simulink library "HEV_Electrical_Lib"  (R2024b)
settings: Solver=ode23t  StartTime=0.0  StopTime=10  MaxStep=1e-3  RelTol=1e-3
values from neighbouring files (symbols this model uses):
  Ts = 2e-6    (= 2e-06)    [param.m]
undefined symbols (not defined in the file or in its folder): DiscIntNeverNeededParam, HEV_Param, magnitude
libraries: fl_lib x73, nesl_utility x30, spsCurrentMeasurementLib x23, spsIdealSwitchLib x12, spsVoltageMeasurementLib x11, simulink_extras x8, spsControlledCurrentSourceLib x7, spsSeriesRLCBranchLib x6, simulink x6, spsControlledVoltageSourceLib x5, spsPermanentMagnetSynchronousMachineLib x4, spsUniversalBridgeLib x3
(part 1 of 4)
Description:
  | Copyright 2008-2023 The MathWorks(TM), Inc.
settings Model: Creator=Xpatrice  LastModifiedBy=froshoo
settings SolverCC: AlgebraicLoopSolver=TrustRegion
settings DataIOCC: LimitDataPoints=on  SaveFormat=Array  SignalLoggingSaveFormat=ModelDataLogs  ReturnWorkspaceOutputs=off
settings OptimizationCC: BlockReduction=off  BooleanDataType=off  ReuseModelBlockBuffer=off  ExpressionDepthLimit=2147483647  LifeSpan=inf
settings DebuggingCC: SaveWithParameterizedLinksMsg=none  UnderspecifiedInitializationDetection=Classic  MergeDetectMultiDrivingBlocksExec=none  SignalResolutionControl=TryResolveAllWithWarning  FcnCallInpInsideContextMsg=warning  UnconnectedInputMsg=warning  UnconnectedOutputMsg=warning  UnconnectedLineMsg=warning  AllowSymbolicDim=off  StateNameClashWarn=warning  PregeneratedLibrarySubsystemCodeDiagnostic=none  SFUnexpectedBacktrackingDiag=warning  SFNoUnconditionalDefaultTransitionDiag=warning  SFExecutionAtInitializationDiag=none  ArithmeticOperatorsInVariantConditions=warning
settings HardwareCC: ProdBitPerPointer=32  ProdBitPerSizeT=32  ProdBitPerPtrDiffT=32  ProdLargestAtomicFloat=None  ProdIntDivRoundTo=Undefined  ProdEndianess=Unspecified  ProdWordSize=32  ProdHWDeviceType=32-bit Generic  TargetUnknown=on
settings ModelReferenceCC: EnableRefExpFcnMdlSchedulingChecks=on  PropagateSignalLabelsOutOfModel=off
settings SFSimCC: SimUseLocalCustomCode=off  CustomCodeUndefinedFunction=UseInterfaceOnly
settings RTWCC: RTWUseLocalCustomCode=off  GPUComputeCapability=3.5  DLArmComputeVersion=19.05
settings CodeAppCC: StateflowObjectComments=on
settings GRTTargetCC: TargetLangStandard=C89/C90 (ANSI)  CombineOutputUpdateFcns=off  GRTInterface=on
settings ConfigComp: CovMetricSettings=dw  CovSaveCumulativeToWorkspaceVar=on  CovSaveSingleToWorkspaceVar=on  CovExternalEMLEnable=off  CovSFcnEnable=off

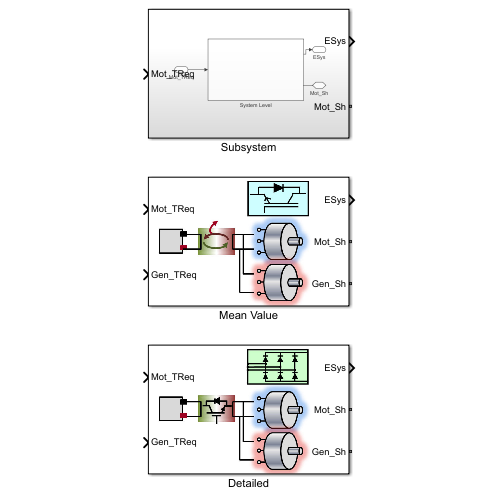
[thumbnail: Simulink's stored preview of the top-level diagram]
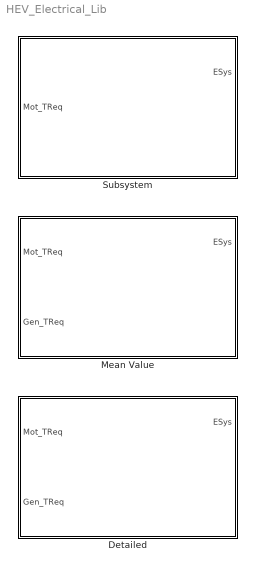
== system HEV_Electrical_Lib ==
  Detailed : Subsystem  mask{popup_batteryvariant=Predefined}
      mask prompts: popup_batteryvariant "Battery Model"
      mask init:
      | set_param([gcb '/Battery'],'LabelModeActiveChoice',get_param(gcb,'popup_batteryvariant'));
      mask TypeOptions popup_batteryvariant: Predefined | Generic
      mask Display: image('HEV_Electrical_Detailed_IMAGE.jpg');
  Mean Value : Subsystem  mask{popup_batteryvariant=Predefined}
      mask prompts: popup_batteryvariant "Battery Model"
      mask init:
      | set_param([gcb '/Battery'],'LabelModeActiveChoice',get_param(gcb,'popup_batteryvariant'));
      mask TypeOptions popup_batteryvariant: Predefined | Generic
      mask Display: image('HEV_Electrical_Mean_Value_IMAGE.jpg');
  Subsystem : Subsystem

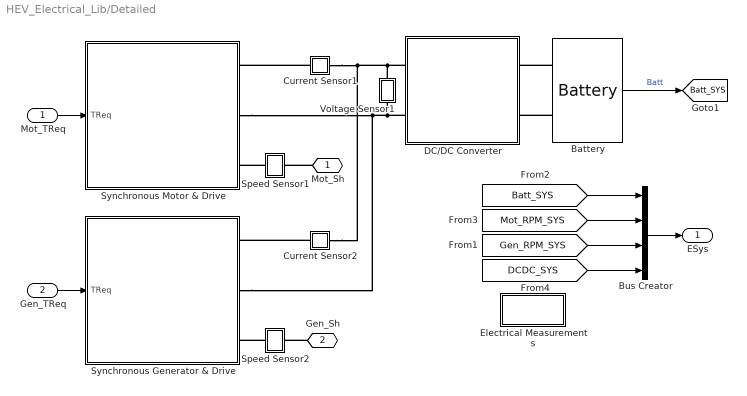
== system HEV_Electrical_Lib/Detailed ==
  Mot_TReq : Inport
  Gen_TReq : Inport  Port=2
  Battery : HEV_Battery_Det_Lib/Battery  SystemSampleTime=-1  LabelModeActiveChoice=Predefined  VariantActivationTime=update diagram  AllowFlexibleInterface=on  Latency=0  AutoFrameSizeCalculation=off
  Bus Creator : BusCreator  Inputs='Batt','Mot_RPM','Gen_RPM','DCDC_Temp'
  Current Sensor1 : Subsystem
  Current Sensor2 : Subsystem
  DC/DC Converter : Subsystem
      mask Display:
      | image(imread('HEV_DCDC_Switching_IMAGE.jpg'));
      | port_label('RConn',1,'Bus+');
      | port_label('RConn',2,'Bus-');
      | port_label('LConn',1,'Batt+');
      | port_label('LConn',2,'Batt-');
      | text(0.05,0.5,'Out');
      | text(0.85,0.5,'In');
  Electrical Measurements : Subsystem
  Speed Sensor1 : Subsystem
      mask Display: disp('S');
  Speed Sensor2 : Subsystem
      mask Display: disp('S');
  Synchronous Generator & Drive : Subsystem
      mask Display:
      | image(imread('HEV_Detailed_Generator_IMAGE.jpg'));
      | port_label('input',1,'T_Req');
      | port_label('RConn',1,'+');
      | port_label('RConn',2,'-');
      | port_label('RConn',3,'Shaft');
  Synchronous Motor & Drive : Subsystem
      mask Display:
      | image(imread('HEV_Detailed_Motor_IMAGE.jpg'));
      | port_label('input',1,'T_Req');
      | port_label('RConn',1,'+');
      | port_label('RConn',2,'-');
      | port_label('RConn',3,'Shaft');
  Voltage Sensor1 : Subsystem
  Mot_Sh : PMIOPort  Side=Right
  Gen_Sh : PMIOPort  Port=2  Side=Right
  ESys : Outport  VectorParamsAs1DForOutWhenUnconnected=off
  tag scope: Batt_SYS=global
  wires:
  [DCDC_SYS] -> Bus Creator/4
  [Batt_SYS] -> Bus Creator/1
  Bus Creator/1 -> ESys/1
  [Gen_RPM_SYS] -> Bus Creator/3
  [Mot_RPM_SYS] -> Bus Creator/2
  Gen_TReq/1 -> Synchronous Generator & Drive/1(TReq)
  Battery/1 -> [Batt_SYS]  "Batt"
  Mot_TReq/1 -> Synchronous Motor & Drive/1(TReq)
  connections:
  Gen_Sh/RConn1 -- Speed Sensor2/RConn1
  Speed Sensor2/LConn1 -- Synchronous Generator & Drive/RConn3
  Mot_Sh/RConn1 -- Speed Sensor1/RConn1
  Speed Sensor1/LConn1 -- Synchronous Motor & Drive/RConn3
  Current Sensor1/LConn1 -- Synchronous Motor & Drive/RConn1
  Current Sensor2/LConn1 -- Synchronous Generator & Drive/RConn1
  Battery/LConn2 -- DC/DC Converter/LConn2
  Battery/LConn1 -- DC/DC Converter/LConn1
  DC/DC Converter/RConn1 -- Current Sensor2/RConn1 -- Current Sensor1/RConn1 -- Voltage Sensor1/RConn1
  DC/DC Converter/RConn2 -- Synchronous Motor & Drive/RConn2 -- Synchronous Generator & Drive/RConn2 -- Voltage Sensor1/LConn1

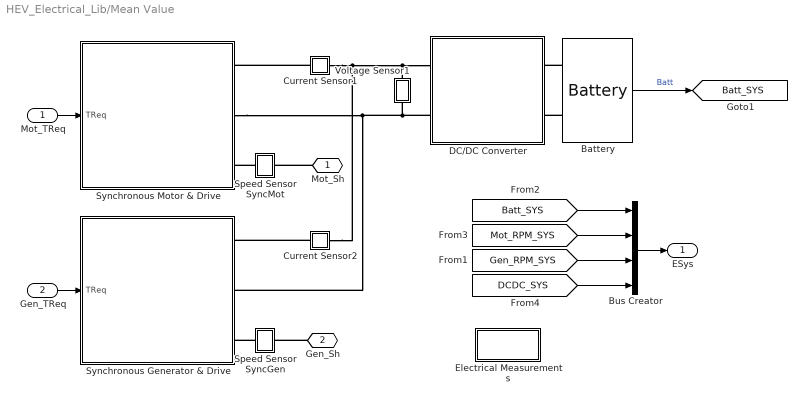
== system HEV_Electrical_Lib/Mean Value ==
  Mot_TReq : Inport
  Gen_TReq : Inport  Port=2
  Battery : HEV_Battery_Det_Lib/Battery  SystemSampleTime=-1  LabelModeActiveChoice=Predefined  VariantActivationTime=update diagram  AllowFlexibleInterface=on  Latency=0  AutoFrameSizeCalculation=off
  Bus Creator : BusCreator  Inputs='Batt','Mot_RPM','Gen_RPM','DCDC_Temp'
  Current Sensor1 : Subsystem
  Current Sensor2 : Subsystem
  DC/DC Converter : Subsystem
      mask init:
      | [X1,X1m,X2,X2m,X3,X4,Y1,Y1m,Y2,Y2m,Y3,Y4,color1,color2]=spsdrivelogo;
      mask Display:
      | image(imread('HEV_DCDC_System_IMAGE.jpg'));
      | port_label('RConn',1,'Bus+');
      | port_label('RConn',2,'Bus-');
      | port_label('LConn',1,'Batt+');
      | port_label('LConn',2,'Batt-');
      | text(0.05,0.5,'Out');
      | text(0.85,0.5,'In');
      | text(0.4,0.925,'Loss');
  Electrical Measurements : Subsystem
  Speed Sensor SyncGen : Subsystem
      mask Display: disp('S');
  Speed Sensor SyncMot : Subsystem
      mask Display: disp('S');
  Synchronous Generator & Drive : Subsystem
      mask Display:
      | image(imread('HEV_MeanValue_Generator_IMAGE.jpg'));
      | port_label('input',1,'T_Req');
      | port_label('RConn',1,'+');
      | port_label('RConn',2,'-');
      | port_label('RConn',3,'Shaft');
  Synchronous Motor & Drive : Subsystem
      mask Display:
      | image(imread('HEV_MeanValue_Motor_IMAGE.jpg'));
      | port_label('input',1,'T_Req');
      | port_label('RConn',1,'+');
      | port_label('RConn',2,'-');
      | port_label('RConn',3,'Shaft');
  Voltage Sensor1 : Subsystem
  Mot_Sh : PMIOPort  Side=Right
  Gen_Sh : PMIOPort  Port=2  Side=Right
  ESys : Outport  VectorParamsAs1DForOutWhenUnconnected=off
  tag scope: Batt_SYS=global
  wires:
  [DCDC_SYS] -> Bus Creator/4
  [Batt_SYS] -> Bus Creator/1
  Bus Creator/1 -> ESys/1
  [Gen_RPM_SYS] -> Bus Creator/3
  [Mot_RPM_SYS] -> Bus Creator/2
  Gen_TReq/1 -> Synchronous Generator & Drive/1(TReq)
  Battery/1 -> [Batt_SYS]  "Batt"
  Mot_TReq/1 -> Synchronous Motor & Drive/1(TReq)
  connections:
  Gen_Sh/RConn1 -- Speed Sensor SyncGen/RConn1
  Speed Sensor SyncGen/LConn1 -- Synchronous Generator & Drive/RConn3
  Mot_Sh/RConn1 -- Speed Sensor SyncMot/RConn1
  Speed Sensor SyncMot/LConn1 -- Synchronous Motor & Drive/RConn3
  Battery/LConn2 -- DC/DC Converter/LConn2
  Battery/LConn1 -- DC/DC Converter/LConn1
  Current Sensor2/RConn1 -- Current Sensor1/RConn1 -- DC/DC Converter/RConn1 -- Voltage Sensor1/RConn1
  DC/DC Converter/RConn2 -- Synchronous Generator & Drive/RConn2 -- Synchronous Motor & Drive/RConn2 -- Voltage Sensor1/LConn1
  Current Sensor1/LConn1 -- Synchronous Motor & Drive/RConn1
  Current Sensor2/LConn1 -- Synchronous Generator & Drive/RConn1

== system HEV_Electrical_Lib/Subsystem ==
  Mot_TReq : Inport
  System Level : Subsystem  mask{popup_batteryvariant=Predefined}
      mask prompts: popup_batteryvariant "Battery Variant"
      mask init:
      | set_param([gcb '/Battery'],'LabelModeActiveChoice',get_param(gcb,'popup_batteryvariant'));
      mask TypeOptions popup_batteryvariant: Predefined | Generic | Cells
      mask Display: image('HEV_Electrical_System_Level_IMAGE.jpg');
  Mot_Sh : PMIOPort  Side=Right
  ESys : Outport
  wires:
  Mot_TReq/1 -> System Level/1(Mot_TReq)
  System Level/1(ESys) -> ESys/1
  connections:
  System Level/RConn1 -- Mot_Sh/RConn1

== system HEV_Electrical_Lib/Detailed/Current Sensor1 ==
  i1 : spsCurrentMeasurementLib/Current Measurement  PhasorSimulation=off  OutputType=Complex  PSBequivalent=0
  - : PMIOPort  Side=Left
  + : PMIOPort  Tag=PMCPort  Port=2  Side=Right
  tag scope: Mot_Current_SYS=global
  wires:
  i1/1 -> [Mot_Current_SYS]
  connections:
  -/RConn1 -- i1/RConn1
  +/RConn1 -- i1/LConn1

== system HEV_Electrical_Lib/Detailed/Current Sensor2 ==
  i1 : spsCurrentMeasurementLib/Current Measurement  PhasorSimulation=off  OutputType=Complex  PSBequivalent=0
  + : PMIOPort  Side=Right
  - : PMIOPort  Port=2  Side=Left
  tag scope: Gen_Current_SYS=global
  wires:
  i1/1 -> [Gen_Current_SYS]
  connections:
  +/RConn1 -- i1/LConn1
  -/RConn1 -- i1/RConn1

== system HEV_Electrical_Lib/Detailed/DC//DC Converter ==
  CBus : spsSeriesRLCBranchLib/Series RLC Branch  LConnTagsString=__new0  RConnTagsString=__new0  BranchType=RC  Resistance=0.1  Inductance=1e-3  SetiL0=off  InitialCurrent=0  Capacitance=1130e-6  Setx0=on  InitialVoltage=500  Measurements=None
  CBus1 : spsSeriesRLCBranchLib/Series RLC Branch  LConnTagsString=__new0  RConnTagsString=__new0  BranchType=C  Resistance=0.2  Inductance=1e-3  SetiL0=off  InitialCurrent=0  Capacitance=282e-6  Setx0=on  InitialVoltage=150  Measurements=None
  Detailed Boost converter : spsUniversalBridgeLib/Universal Bridge  Arms=1  SnubberResistance=5000  SnubberCapacitance=inf  Device=IGBT / Diodes  Ron=1e-3  Lon=0  ForwardVoltages=[0,0]  ForwardVoltage=0  GTOparameters=[ 10e-6 , 20e-6 ]  IGBTparameters=[0,0]  Measurements=None  Measurements_2=None  converterType=Rectifier
  L : spsSeriesRLCBranchLib/Series RLC Branch  LConnTagsString=__new0  RConnTagsString=__new0  BranchType=L  Resistance=0.3  Inductance=373e-6  SetiL0=off  InitialCurrent=100  Capacitance=100e-6  Setx0=off  InitialVoltage=0  Measurements=None
  PWM : Subsystem
  Ubus Ref : Constant  Value=HEV_Param.DCDCConv.Output_Voltage
  V1 : spsVoltageMeasurementLib/Voltage Measurement  PhasorSimulation=off  OutputType=Complex  PSBequivalent=0
  Voltage Controller : Subsystem  mask(PI controller){Kp=0.001, Ki=1, Ts=Ts}
      mask prompts: Kp "Proportional gain (Kp)"; Ki "Integral gain (Ki)"; Ts "Sample time (s) :"
      mask help: Proportional-Integral Speed Controller
      mask Display: plot(0,0,100,100,[35,35,65],[70,30,30],[35,65],[45,60])
  Bus+ : PMIOPort  Tag=PMCPort  Side=Right
  Bus- : PMIOPort  Tag=PMCPort  Port=2  Side=Right
  Batt+ : PMIOPort  Tag=PMCPort  Port=3  Side=Left
  Batt- : PMIOPort  Tag=PMCPort  Port=4  Side=Left
  wires:
  PWM/1(Pulses) -> Detailed Boost converter/1
  Voltage Controller/1(Ec) -> PWM/1(Ref.)
  Ubus Ref/1 -> Voltage Controller/1(Uref)
  V1/1 -> Voltage Controller/2(UBus)
  connections:
  L/LConn1 -- Detailed Boost converter/LConn1
  Detailed Boost converter/RConn1 -- CBus/LConn1 -- V1/LConn1 -- Bus+/RConn1
  Batt+/RConn1 -- L/RConn1 -- CBus1/LConn1
  Detailed Boost converter/RConn2 -- Bus-/RConn1 -- CBus/RConn1 -- V1/LConn2 -- Batt-/RConn1 -- CBus1/RConn1

== system HEV_Electrical_Lib/Detailed/Electrical Measurements ==
  Bus Selector : BusSelector  OutputSignals=Voltage (V),Current (A),SOC (%)
  Mux : Mux  Inputs=2
  Mux1 : Mux  Inputs=3
  Mux2 : Mux  Inputs=3
  Mux3 : Mux
  Mux4 : Mux  Inputs=2
  Product1 : Product  RndMeth=Zero
  Product2 : Product  RndMeth=Zero
  Product3 : Product  RndMeth=Zero
  tag scope: Electricals=global, Power=global
  wires:
  Product2/1 -> Mux1/1  "Motor Power (W)"
  Product1/1 -> Mux1/2  "Generator power (W)"
  Product3/1 -> Mux1/3  "Battery power (W)"
  [Mot_Current_SYS] -> Product2/1, Mux2/1
  Mux1/1 -> [Power]
  [Batt_Measures] -> Bus Selector/1
  Bus Selector/1 -> Mux/2, Product3/1  "<Voltage (V)>"
  Bus Selector/2 -> Product3/2, Mux2/2  "<Current (A)>"
  Mux/1 -> Mux3/2  "Voltage (DC bus, Battery)"
  Mux2/1 -> Mux3/3  "Current (Motor, Battery, Generator)"
  [Gen_Current_SYS] -> Product1/1, Mux2/3
  Bus Selector/3 -> Mux3/4  "<SOC (%)>"
  [DC_Bus_SYS] -> Product2/2, Product1/2, Mux/1, Mux4/1, Mux4/2
  Mux3/1 -> [Electricals]
  Mux4/1 -> Mux3/1

== system HEV_Electrical_Lib/Detailed/Speed Sensor1 ==
  Ideal Rotational Motion Sensor : fl_lib/Mechanical/Mechanical Sensors/Ideal Rotational Motion Sensor  reference=foundation.enum.MeasurementReference.difference  acceleration_port=false  velocity_port=true  position_port=true  wrap_angle=simscape.enum.onoff.off  offset=0 rad
  Mechanical Rotational Reference : fl_lib/Mechanical/Rotational Elements/Mechanical Rotational Reference
  PS-Simulink Converter : nesl_utility/PS-Simulink Converter  PhysicalDomain=network_engine_domain  SubClassName=ps_output  LeftPortType=input  RightPortType=output  PseudoPeriodic=off  Frequencies=[]  VectorFormat=1-D array  Unit=rpm  AffineConversion=off
  Solver Configuration : nesl_utility/Solver Configuration  PhysicalDomain=network_engine_domain  SubClassName=solver  LeftPortType=input  RightPortType=generic  Tones=[]  Harmonics=[]  SimulateNoise=off  Profile=off  UseLocalSampling=off  EnableSwitchedLinearOptims=on  FrequencyDomain=off  UseCCode=off  RelTol=0.001  AbsTol=0.001  MinStep=1e-09  ToWorkspace=off  RevertToSquareIcSolve=off  NumHomotopyIterations=100  PhasorMode=off  PhasorModeNumHarmonics=1  ConsistencySolver=NEWTON_XTOL_AFTER_FTOL  IndexReductionMethod=DerivativeReplacement  DoDC=off  ResidualTolerance=1e-09  ConsistencyTolSource=GLOBAL  ConsistencyAbsTol=0.001  ConsistencyRelTol=0.001  ConsistencyTolFactor=0.001  UseLocalSolver=off  LocalSolverChoice=NE_BACKWARD_EULER_ADVANCER  ResolveIndetEquations=on  FunctionEvalNumThread=1  LocalSolverSampleTime=0.001  DoFixedCost=off  MaxNonlinIter=3  MaxModeIter=2  ComputeImpulses=off  ImpulseIterations=2  LinearAlgebra=auto  LinearAlgebraNumThread=0  EquationFormulation=NE_TIME_EF  DelaysMemoryBudget=1024  AutomaticFiltering=on  FilteringTimeConstant=0.001  PartitionStorageMethod=AS_NEEDED  PartitionMemoryBudget=1024  PartitionMethod=ROBUST  MultibodyUseLocalSolver=off  MultibodyLocalSolverChoice=ODE1  MultibodyLocalSolverSampleTime=0.001
  Sh : PMIOPort  Side=Left
  Sh1 : PMIOPort  Port=2  Side=Right
  tag scope: Mot_RPM_SYS=global
  wires:
  PS-Simulink Converter/1 -> [Mot_RPM_SYS]  "Mot_RPM"
  connections:
  Ideal Rotational Motion Sensor/RConn1 -- Mechanical Rotational Reference/LConn1
  Sh1/RConn1 -- Solver Configuration/RConn1 -- Ideal Rotational Motion Sensor/LConn1 -- Sh/RConn1
  PS-Simulink Converter/LConn1 -- Ideal Rotational Motion Sensor/RConn2

== system HEV_Electrical_Lib/Detailed/Speed Sensor2 ==
  Ideal Rotational Motion Sensor : fl_lib/Mechanical/Mechanical Sensors/Ideal Rotational Motion Sensor  reference=foundation.enum.MeasurementReference.difference  acceleration_port=false  velocity_port=true  position_port=true  wrap_angle=simscape.enum.onoff.off  offset=0 rad
  Mechanical Rotational Reference : fl_lib/Mechanical/Rotational Elements/Mechanical Rotational Reference
  PS-Simulink Converter : nesl_utility/PS-Simulink Converter  PhysicalDomain=network_engine_domain  SubClassName=ps_output  LeftPortType=input  RightPortType=output  PseudoPeriodic=off  Frequencies=[]  VectorFormat=1-D array  Unit=rpm  AffineConversion=off
  Solver Configuration : nesl_utility/Solver Configuration  PhysicalDomain=network_engine_domain  SubClassName=solver  LeftPortType=input  RightPortType=generic  Tones=[]  Harmonics=[]  SimulateNoise=off  Profile=off  UseLocalSampling=off  EnableSwitchedLinearOptims=on  FrequencyDomain=off  UseCCode=off  RelTol=0.001  AbsTol=0.001  MinStep=1e-09  ToWorkspace=off  RevertToSquareIcSolve=off  NumHomotopyIterations=100  PhasorMode=off  PhasorModeNumHarmonics=1  ConsistencySolver=NEWTON_XTOL_AFTER_FTOL  IndexReductionMethod=DerivativeReplacement  DoDC=off  ResidualTolerance=1e-09  ConsistencyTolSource=GLOBAL  ConsistencyAbsTol=0.001  ConsistencyRelTol=0.001  ConsistencyTolFactor=0.001  UseLocalSolver=off  LocalSolverChoice=NE_BACKWARD_EULER_ADVANCER  ResolveIndetEquations=on  FunctionEvalNumThread=1  LocalSolverSampleTime=0.001  DoFixedCost=off  MaxNonlinIter=3  MaxModeIter=2  ComputeImpulses=off  ImpulseIterations=2  LinearAlgebra=auto  LinearAlgebraNumThread=0  EquationFormulation=NE_TIME_EF  DelaysMemoryBudget=1024  AutomaticFiltering=on  FilteringTimeConstant=0.001  PartitionStorageMethod=AS_NEEDED  PartitionMemoryBudget=1024  PartitionMethod=ROBUST  MultibodyUseLocalSolver=off  MultibodyLocalSolverChoice=ODE1  MultibodyLocalSolverSampleTime=0.001
  Sh : PMIOPort  Side=Left
  Sh1 : PMIOPort  Port=2  Side=Right
  tag scope: Gen_RPM_SYS=global
  wires:
  PS-Simulink Converter/1 -> [Gen_RPM_SYS]  "Gen_RPM"
  connections:
  Ideal Rotational Motion Sensor/RConn1 -- Mechanical Rotational Reference/LConn1
  PS-Simulink Converter/LConn1 -- Ideal Rotational Motion Sensor/RConn2
  Sh1/RConn1 -- Sh/RConn1 -- Solver Configuration/RConn1 -- Ideal Rotational Motion Sensor/LConn1

== system HEV_Electrical_Lib/Detailed/Synchronous Generator & Drive ==
  note: This block is based on the AC6
      | drive block
  TReq : Inport
  Bus Selector : BusSelector  OutputSignals=Rotor angle thetam (rad)
  GF : Subsystem
      mask Display: disp('GF')
  Measures : Subsystem
      settings: LibrarySourceBlock=electricdrivelib/AC drives/PM Synchronous Motor Drive/Measures
  Mux : Subsystem
  Permanent Magnet Synchronous Machine : spsPermanentMagnetSynchronousMachineLib/Permanent Magnet Synchronous Machine  NbPhases=3  FluxDistribution=Sinusoidal  RotorType=Salient-pole  MechanicalLoad=Speed w  PresetModel=No  ShowDetailedParameters=on  MeasurementBus=off  Resistance=HEV_Param.Generator.Stator_Resistance  Inductance=0  dqInductances=HEV_Param.Generator.Inductances  La=0.000835  MachineConstant=Flux linkage established by magnets (V.s)  Flux=0.192  VoltageCst=34.8249  TorqueCst=0.288  Flat=0  Mechanical=[0.011 0.001889/4 4/4]  PolePairs=1  InitialConditions=[0,0, 0,0,0]  InitialConditions5ph=[0 0 0 0 0 0]  RefAngle=90 degrees behind phase A axis (modified Park)  IterativeDiscreteModel=Trapezoidal non iterative  TsBlock=-1  TsPowergui=0
      settings: AttributesFormatString=\n
  Shaft Inertia : fl_lib/Mechanical/Rotational Elements/Inertia  inertia=HEV_Param.Generator.Shaft_Inertia kg*m^2  num_ports=foundation.enum.numPorts2.one  w_specify=on  w_priority=High  w=0 rad/s  w_nominal_specify=off  w_nominal_value=1  w_nominal_unit=rad/s  t_specify=off  t_priority=High  t=0 N*m  t_nominal_specify=off  t_nominal_value=1  t_nominal_unit=N*m
  Subsystem : Subsystem
      mask Display: disp('GF');
  Subsystem1 : Subsystem
  Three-phase Inverter : spsUniversalBridgeLib/Universal Bridge  Arms=3  SnubberResistance=5000  SnubberCapacitance=inf  Device=IGBT / Diodes  Ron=1e-3  Lon=0  ForwardVoltages="[  0  0  ]"  ForwardVoltage=0  GTOparameters=[ 10e-6 , 20e-6 ]  IGBTparameters=[ 1e-6 , 2e-6 ]*0  Measurements=None  Measurements_2=None  converterType=Rectifier
  VECT : Subsystem  mask(VECT){nb_p=1, lambda=0.192, freq_max=20e3, Ts_vect=20e-6, h=0.1}
      mask prompts: nb_p "Motor pairs of poles"; lambda "Flux induced by magnets (Wb)"; freq_max "Maximum switching frequency (Hz)"; Ts_vect "Sampling time (s)"; h "Current hysteresis bandwidth (A)"
      mask help: This block implements a vector controller.
      mask init:
      | load spsdrivelogodata.mat
      mask Display:
      | patch([spsdrivelogodata.X1 spsdrivelogodata.X1m],[spsdrivelogodata.Y1 spsdrivelogodata.Y1m],spsdrivelogodata.color1);
      | patch(spsdrivelogodata.X3,spsdrivelogodata.Y3,spsdrivelogodata.color2);
      | plot([spsdrivelogodata.X1 spsdrivelogodata.X1m spsdrivelogodata.X2 spsdrivelogodata.X2m spsdrivelogodata.X3 spsdrivelogodata.X4],[spsdrivelogodata.Y1 spsdrivelogodata.Y1m spsdrivelogodata.Y2 spsdrivelogodata.Y2m spsdrivelogodata.Y3 spsdrivelogodata.Y4]);
  + : PMIOPort  Side=Right
  - : PMIOPort  Port=2  Side=Right
  Gen_Sh : PMIOPort  Port=3  Side=Right
  wires:
  TReq/1 -> GF/1(In1)
  Bus Selector/1 -> VECT/2(teta)  "<Rotor angle thetam (rad)>"
  Mux/1(g) -> Three-phase Inverter/1
  VECT/1(gates) -> Mux/1(gates)
  Measures/1(I_abc) -> VECT/3(I_abc)
  Permanent Magnet Synchronous Machine/1 -> Bus Selector/1, Mux/2(m), Subsystem/1(In)
  Subsystem/1(Out) -> Subsystem1/1(Sig)
  Subsystem1/1(Spd) -> Permanent Magnet Synchronous Machine/1
  GF/1(Out1) -> VECT/1(Torque*)
  connections:
  Three-phase Inverter/LConn3 -- Measures/LConn3
  Measures/LConn2 -- Three-phase Inverter/LConn2
  Three-phase Inverter/LConn1 -- Measures/LConn1
  Measures/RConn3 -- Permanent Magnet Synchronous Machine/LConn3
  Measures/RConn2 -- Permanent Magnet Synchronous Machine/LConn2
  Measures/RConn1 -- Permanent Magnet Synchronous Machine/LConn1
  +/RConn1 -- Three-phase Inverter/RConn1
  -/RConn1 -- Three-phase Inverter/RConn2
  Subsystem1/RConn1 -- Gen_Sh/RConn1 -- Shaft Inertia/LConn1

== system HEV_Electrical_Lib/Detailed/Synchronous Motor & Drive ==
  note: This block is based on the
      | AC6 IPMSM drive block
  TReq : Inport
  500 Vdc 50kW PMSM : spsPermanentMagnetSynchronousMachineLib/Permanent Magnet Synchronous Machine  NbPhases=3  FluxDistribution=Sinusoidal  RotorType=Salient-pole  MechanicalLoad=Speed w  PresetModel=No  ShowDetailedParameters=on  MeasurementBus=off  Resistance=HEV_Param.Motor.Stator_Resistance  Inductance=0  dqInductances=HEV_Param.Motor.Inductances  La=0.000835  MachineConstant=Flux linkage established by magnets (V.s)  Flux=0.175666143629361  VoltageCst=127.4493  TorqueCst=1.054  Flat=0  Mechanical=[0.089 0.005 4]  PolePairs=4  InitialConditions=[0,0,0,0]  InitialConditions5ph=[0 0 0 0 0 0]  RefAngle=90 degrees behind phase A axis (modified Park)  IterativeDiscreteModel=Trapezoidal non iterative  TsBlock=-1  TsPowergui=0
      settings: AttributesFormatString=\n
  Bus Selector : BusSelector  OutputSignals=Rotor speed wm (rad/s),Rotor angle thetam (rad)
  GF : Subsystem
      mask Display: disp('GF')
  Measures : Subsystem
      settings: LibrarySourceBlock=electricdrivelib/AC drives/PM Synchronous Motor Drive/Measures
  Mux : Subsystem
  Shaft Inertia : fl_lib/Mechanical/Rotational Elements/Inertia  inertia=HEV_Param.Motor.Shaft_Inertia kg*m^2  num_ports=foundation.enum.numPorts2.one  w_specify=on  w_priority=High  w=0 rad/s  w_nominal_specify=off  w_nominal_value=1  w_nominal_unit=rad/s  t_specify=off  t_priority=High  t=0 N*m  t_nominal_specify=off  t_nominal_value=1  t_nominal_unit=N*m
  Subsystem : Subsystem
      mask Display: disp('GF');
  Subsystem1 : Subsystem
  Three-Phase Inverter : spsUniversalBridgeLib/Universal Bridge  Arms=3  SnubberResistance=5000  SnubberCapacitance=inf  Device=IGBT / Diodes  Ron=1e-3  Lon=0  ForwardVoltages="[  0  0  ]"  ForwardVoltage=0  GTOparameters=[ 10e-6 , 20e-6 ]  IGBTparameters=[ 1e-6 , 2e-6 ]*0  Measurements=None  Measurements_2=None  converterType=Rectifier
  Torque limitation : Subsystem
      mask Display: plot([0;1800;2000;2500;3000;3500], [1;1;0.90*1;0.72*1;0.6*1;0.51*1])
  VECT Controller : Subsystem  mask(VECT){nb_p=4, dqInductances=HEV_Param.Motor.Inductances, lambda=0.175666143629361, freq_max=20e3, Ts_vect=20e-6, h=0.1}
      mask prompts: nb_p "Motor pairs of poles"; dqInductances "Inductances [ Ld(H) Lq(H) ]:"; lambda "Flux induced by magnets (Wb)"; freq_max "Maximum switching frequency (Hz)"; Ts_vect "Sampling time (s)"; h "Current hysteresis bandwidth (A)"
      mask help: This block implements a vector controller.
      mask init:
      | load spsdrivelogodata.mat
      | ib = lambda/(dqInductances(2)-dqInductances(1));
      | Teb = 3/2*nb_p*lambda*ib;
      | Ld = dqInductances(1);
      | Lq = dqInductances(2);
      | lam = lambda;
      | p=nb_p;
      | ib = lam/(Lq-Ld);
      | iqn = 0:0.01:3;
      | ten = iqn/2.*(sqrt(4*iqn.*iqn+1)+1);
      mask Display:
      | patch([spsdrivelogodata.X1 spsdrivelogodata.X1m],[spsdrivelogodata.Y1 spsdrivelogodata.Y1m],spsdrivelogodata.color1);
      | patch(spsdrivelogodata.X3,spsdrivelogodata.Y3,spsdrivelogodata.color2);
      | plot([spsdrivelogodata.X1 spsdrivelogodata.X1m spsdrivelogodata.X2 spsdrivelogodata.X2m spsdrivelogodata.X3 spsdrivelogodata.X4],[spsdrivelogodata.Y1 spsdrivelogodata.Y1m spsdrivelogodata.Y2 spsdrivelogodata.Y2m spsdrivelogodata.Y3 spsdrivelogodata.Y4]);
  + : PMIOPort  Side=Right
  - : PMIOPort  Port=2  Side=Right
  Mot_Sh : PMIOPort  Port=3  Side=Right
  wires:
  TReq/1 -> GF/1(In1)
  Torque limitation/1(torque) -> VECT Controller/1(Torque*)
  Bus Selector/2 -> VECT Controller/3(teta)  "<Rotor angle thetam (rad)>"
  Measures/1(I_abc) -> VECT Controller/4(I_abc)
  Bus Selector/1 -> Torque limitation/1(N rad/s), VECT Controller/2(w)  "<Rotor speed wm (rad/s)>"
  500 Vdc 50kW PMSM/1 -> Bus Selector/1, Mux/2(m), Subsystem/1(In)
  VECT Controller/1(gates) -> Mux/1(gates)
  Mux/1(g) -> Three-Phase Inverter/1
  Subsystem/1(Out) -> Subsystem1/1(Sig)
  Subsystem1/1(Spd) -> 500 Vdc 50kW PMSM/1
  GF/1(Out1) -> Torque limitation/2(Torque)
  connections:
  -/RConn1 -- Three-Phase Inverter/RConn2
  +/RConn1 -- Three-Phase Inverter/RConn1
  Measures/RConn1 -- 500 Vdc 50kW PMSM/LConn1
  Measures/RConn2 -- 500 Vdc 50kW PMSM/LConn2
  Measures/RConn3 -- 500 Vdc 50kW PMSM/LConn3
  Three-Phase Inverter/LConn1 -- Measures/LConn1
  Measures/LConn2 -- Three-Phase Inverter/LConn2
  Three-Phase Inverter/LConn3 -- Measures/LConn3
  Shaft Inertia/LConn1 -- Mot_Sh/RConn1 -- Subsystem1/RConn1

== system HEV_Electrical_Lib/Detailed/Voltage Sensor1 ==
  V1 : spsVoltageMeasurementLib/Voltage Measurement  PhasorSimulation=off  OutputType=Complex  PSBequivalent=0
  + : PMIOPort  Tag=PMCPort  Side=Right
  - : PMIOPort  Port=2  Side=Left
  tag scope: DC_Bus_SYS=global
  wires:
  V1/1 -> [DC_Bus_SYS]
  connections:
  +/RConn1 -- V1/LConn1
  -/RConn1 -- V1/LConn2

== system HEV_Electrical_Lib/Mean Value/Current Sensor1 ==
  i1 : spsCurrentMeasurementLib/Current Measurement  PhasorSimulation=off  OutputType=Complex  PSBequivalent=0
  - : PMIOPort  Side=Left
  + : PMIOPort  Tag=PMCPort  Port=2  Side=Right
  tag scope: Mot_Current_SYS=global
  wires:
  i1/1 -> [Mot_Current_SYS]
  connections:
  -/RConn1 -- i1/RConn1
  +/RConn1 -- i1/LConn1

== system HEV_Electrical_Lib/Mean Value/Current Sensor2 ==
  i1 : spsCurrentMeasurementLib/Current Measurement  PhasorSimulation=off  OutputType=Complex  PSBequivalent=0
  + : PMIOPort  Side=Right
  - : PMIOPort  Port=2  Side=Left
  tag scope: Gen_Current_SYS=global
  wires:
  i1/1 -> [Gen_Current_SYS]
  connections:
  +/RConn1 -- i1/LConn1
  -/RConn1 -- i1/RConn1

== system HEV_Electrical_Lib/Mean Value/DC//DC Converter ==
  Boost Converter Average-Values : Subsystem  mask(SPSdrives Converter){SnubberResistance=10e3, SnubberCapacitance=inf, Ron=1e-3, ForwardVoltages=[1.3,1.3], IGBTParameters=[0,0], converterType=Inverter}
      mask prompts: SnubberResistance "Snubber resistance Rs (Ohms):"; SnubberCapacitance "Snubber capacitance Cs (F):"; Ron "Ron (Ohms):"; ForwardVoltages "Forward voltages [Device Vf(V), Diode Vd (V)]"; IGBTParameters "[Tf(s), Tt(s)]:"; converterType "Converter type:"
      mask help: This model implements an average-value buck converter."Duty Cycle" contains the duty cycle of the internal IGBT device.
      mask TypeOptions converterType: Rectifier | Inverter
      mask Display: plot(0,0,100,100,[39 39 23.8],[71 28 28],[44 56 49.6 56 52.8 56 61 61],[39.2 33.6 32.8 33.6 40.8 33.6 30 12.4],[44 44 44 61 61],[28 71 60 66.4 90],[75 67 83 75 67 83 75 75],[54 42 42 54 54 54 54 66],[61 75 75],[24 24 42],[75 75 61],[66,76,76])
  CBus : spsSeriesRLCBranchLib/Series RLC Branch  LConnTagsString=__new0  RConnTagsString=__new0  BranchType=RC  Resistance=0.1  Inductance=1e-3  SetiL0=off  InitialCurrent=0  Capacitance=1130e-6  Setx0=on  InitialVoltage=500  Measurements=None
  CBus1 : spsSeriesRLCBranchLib/Series RLC Branch  LConnTagsString=__new0  RConnTagsString=__new0  BranchType=C  Resistance=0.2  Inductance=1e-3  SetiL0=off  InitialCurrent=0  Capacitance=282e-6  Setx0=on  InitialVoltage=150  Measurements=None
  Current controller DISCRETE3 : Subsystem  mask(PI controller){Kp=HEV_Param.DCDCConv.Mean_Boost.Kp, Ki=HEV_Param.DCDCConv.Mean_Boost.Ki, Ts=Ts}
      mask prompts: Kp "Proportional gain (Kp)"; Ki "Integral gain (Ki)"; Ts "Sample time (s) :"
      mask help: Proportional-Integral Speed Controller
      mask Display: plot(0,0,100,100,[35,35,65],[70,30,30],[35,65],[45,60])
  Duty Cycles : Subsystem
  L : spsSeriesRLCBranchLib/Series RLC Branch  LConnTagsString=__new0  RConnTagsString=__new0  BranchType=L  Resistance=0.3  Inductance=373e-6  SetiL0=off  InitialCurrent=100  Capacitance=100e-6  Setx0=off  InitialVoltage=0  Measurements=None
  Ubus Ref : Constant  Value=HEV_Param.DCDCConv.Output_Voltage
  V1 : spsVoltageMeasurementLib/Voltage Measurement  PhasorSimulation=off  OutputType=Complex  PSBequivalent=0
  Bus+ : PMIOPort  Tag=PMCPort  Side=Right
  Bus- : PMIOPort  Tag=PMCPort  Port=2  Side=Right
  Batt+ : PMIOPort  Tag=PMCPort  Port=3  Side=Left
  Batt- : PMIOPort  Tag=PMCPort  Port=4  Side=Left
  wires:
  Duty Cycles/1(dc) -> Boost Converter Average-Values/1(Duty Cycle)
  Current controller DISCRETE3/1(Ec) -> Duty Cycles/1(Ec)
  Ubus Ref/1 -> Current controller DISCRETE3/1(Uref)
  V1/1 -> Current controller DISCRETE3/2(UBus)
  connections:
  L/LConn1 -- Boost Converter Average-Values/RConn1
  Bus+/RConn1 -- Boost Converter Average-Values/LConn1 -- CBus/LConn1 -- V1/LConn1
  Boost Converter Average-Values/LConn2 -- CBus1/RConn1 -- Batt-/RConn1 -- Bus-/RConn1 -- CBus/RConn1 -- V1/LConn2
  CBus1/LConn1 -- Batt+/RConn1 -- L/RConn1

== system HEV_Electrical_Lib/Mean Value/Electrical Measurements ==
  Bus Selector : BusSelector  OutputSignals=Voltage (V),Current (A),SOC (%)
  Mux : Mux  Inputs=2
  Mux1 : Mux  Inputs=3
  Mux2 : Mux  Inputs=3
  Mux3 : Mux
  Mux4 : Mux  Inputs=2
  Product1 : Product  RndMeth=Zero
  Product2 : Product  RndMeth=Zero
  Product3 : Product  RndMeth=Zero
  tag scope: Electricals=global, Power=global
  wires:
  Mux4/1 -> Mux3/1
  Mux3/1 -> [Electricals]
  [DC_Bus_SYS] -> Mux4/2, Mux4/1, Mux/1, Product1/2, Product2/2
  Bus Selector/3 -> Mux3/4  "<SOC (%)>"
  [Gen_Current_SYS] -> Mux2/3, Product1/1
  Mux2/1 -> Mux3/3  "Current (Motor, Battery, Generator)"
  Mux/1 -> Mux3/2  "Voltage (DC bus, Battery)"
  Bus Selector/2 -> Mux2/2, Product3/2  "<Current (A)>"
  Bus Selector/1 -> Product3/1, Mux/2  "<Voltage (V)>"
  [Batt_Measures] -> Bus Selector/1
  Mux1/1 -> [Power]
  [Mot_Current_SYS] -> Mux2/1, Product2/1
  Product3/1 -> Mux1/3  "Battery power (W)"
  Product1/1 -> Mux1/2  "Generator power (W)"
  Product2/1 -> Mux1/1  "Motor Power (W)"

== system HEV_Electrical_Lib/Mean Value/Speed Sensor SyncGen ==
  Ideal Rotational Motion Sensor : fl_lib/Mechanical/Mechanical Sensors/Ideal Rotational Motion Sensor  reference=foundation.enum.MeasurementReference.difference  acceleration_port=false  velocity_port=true  position_port=true  wrap_angle=simscape.enum.onoff.off  offset=0 rad
  Mechanical Rotational Reference : fl_lib/Mechanical/Rotational Elements/Mechanical Rotational Reference
  PS-Simulink Converter : nesl_utility/PS-Simulink Converter  PhysicalDomain=network_engine_domain  SubClassName=ps_output  LeftPortType=input  RightPortType=output  PseudoPeriodic=off  Frequencies=[]  VectorFormat=1-D array  Unit=rpm  AffineConversion=off
  Sh : PMIOPort  Side=Left
  Sh1 : PMIOPort  Port=2  Side=Right
  tag scope: Gen_RPM_SYS=global
  wires:
  PS-Simulink Converter/1 -> [Gen_RPM_SYS]  "Gen_RPM"
  connections:
  Sh/RConn1 -- Sh1/RConn1 -- Ideal Rotational Motion Sensor/LConn1
  PS-Simulink Converter/LConn1 -- Ideal Rotational Motion Sensor/RConn2
  Ideal Rotational Motion Sensor/RConn1 -- Mechanical Rotational Reference/LConn1

== system HEV_Electrical_Lib/Mean Value/Speed Sensor SyncMot ==
  Ideal Rotational Motion Sensor : fl_lib/Mechanical/Mechanical Sensors/Ideal Rotational Motion Sensor  reference=foundation.enum.MeasurementReference.difference  acceleration_port=false  velocity_port=true  position_port=true  wrap_angle=simscape.enum.onoff.off  offset=0 rad
  Mechanical Rotational Reference : fl_lib/Mechanical/Rotational Elements/Mechanical Rotational Reference
  PS-Simulink Converter : nesl_utility/PS-Simulink Converter  PhysicalDomain=network_engine_domain  SubClassName=ps_output  LeftPortType=input  RightPortType=output  PseudoPeriodic=off  Frequencies=[]  VectorFormat=1-D array  Unit=rpm  AffineConversion=off
  Sh : PMIOPort  Side=Left
  Sh1 : PMIOPort  Port=2  Side=Right
  tag scope: Mot_RPM_SYS=global
  wires:
  PS-Simulink Converter/1 -> [Mot_RPM_SYS]  "Mot_RPM"
  connections:
  PS-Simulink Converter/LConn1 -- Ideal Rotational Motion Sensor/RConn2
  Sh/RConn1 -- Ideal Rotational Motion Sensor/LConn1 -- Sh1/RConn1
  Ideal Rotational Motion Sensor/RConn1 -- Mechanical Rotational Reference/LConn1

== system HEV_Electrical_Lib/Mean Value/Synchronous Generator & Drive ==
  note: This block is based on the AC6
      | drive block
  TReq : Inport
  Bus Selector : BusSelector  OutputSignals=Rotor angle thetam (rad)
  GF : Subsystem
      mask Display: disp('GF')
  Measures : Subsystem
      settings: LibrarySourceBlock=electricdrivelib/AC drives/PM Synchronous Motor Drive/Measures
  Mux : Subsystem
  Permanent Magnet Synchronous Machine : spsPermanentMagnetSynchronousMachineLib/Permanent Magnet Synchronous Machine  NbPhases=3  FluxDistribution=Sinusoidal  RotorType=Salient-pole  MechanicalLoad=Speed w  PresetModel=No  ShowDetailedParameters=on  MeasurementBus=off  Resistance=HEV_Param.Generator.Stator_Resistance  Inductance=0  dqInductances=HEV_Param.Generator.Inductances  La=0.000835  MachineConstant=Flux linkage established by magnets (V.s)  Flux=0.192  VoltageCst=34.8249  TorqueCst=0.288  Flat=0  Mechanical=[0.011 0.001889/4 4/4]  PolePairs=1  InitialConditions=[0,0, 0,0,0]  InitialConditions5ph=[0 0 0 0 0 0]  RefAngle=90 degrees behind phase A axis (modified Park)  IterativeDiscreteModel=Trapezoidal non iterative  TsBlock=-1  TsPowergui=0
      settings: AttributesFormatString=\n
  Shaft Inertia : fl_lib/Mechanical/Rotational Elements/Inertia  inertia=HEV_Param.Generator.Shaft_Inertia kg*m^2  num_ports=foundation.enum.numPorts2.one  w_specify=on  w_priority=High  w=0 rad/s  w_nominal_specify=off  w_nominal_value=1  w_nominal_unit=rad/s  t_specify=off  t_priority=High  t=0 N*m  t_nominal_specify=off  t_nominal_value=1  t_nominal_unit=N*m
  Subsystem : Subsystem
      mask Display: disp('GF');
  Subsystem1 : Subsystem
  Three-phase Inverter : Subsystem  mask(SPSdrives Converter){Arms=3, SnubberResistance=5000, SnubberCapacitance=inf, Device=IGBT / Diodes, Ron=1e-3, Lon=0, ForwardVoltages=[0.8,0.8], ForwardVoltage=0, GTOparameters=[0,0], IGBTparameters=[1e-6,2e-6], Measurements=All voltages and currents, SourceFrequency=60, dqInductances=HEV_Param.Generator.Inductances, Flux=0.192, Resistance=HEV_Param.Generator.Stator_Resistance, p=4/4, converterType=Inverter}
      mask prompts: Arms "Number of bridge arms:"; SnubberResistance "Snubber resistance Rs (Ohms)"; SnubberCapacitance "Snubber capacitance Cs (F)"; Device "Power Electronic device"; Ron "Ron (Ohms)"; Lon "Lon (H)"; ForwardVoltages "Forward voltages  [ Device Vf(V) , Diode Vfd(V)]"; ForwardVoltage "Forward voltage Vf (V)"; GTOparameters "[  Tf (s) , Tt (s)  ]"; IGBTparameters "[  Tf (s) , Tt (s)  ]"; SourceFrequency "Source Frequency (Hz)"; dqInductances "PMSM-Inductances [ Ld(H) Lq(H) ]:"; Flux "PMSM-Flux induced by magnets (Wb):"; Resistance "PMSM-Stator resistance Rs (ohm):"; p "PMSM-Pairs of poles p:"; converterType "Converter type:"
      mask init:
      | Ld=dqInductances(1);
      | Lq=dqInductances(2);
      | Fcs=6*SourceFrequency/10;
      settings: OpenFcn=power_openblockproxy();
      mask Help: web(psbhelp);
      mask TypeOptions Arms: 1 | 2 | 3
      mask TypeOptions Device: Diodes | Thyristors | GTO / Diodes | MOSFET / Diodes | IGBT / Diodes | Ideal Switches
      mask TypeOptions Measurements: None | Device voltages | Device currents | UAB UBC UCA UDC voltages | All voltages and currents
      mask TypeOptions converterType: Rectifier | Inverter
      mask Display: plot(0,0,100,100,[39 39 23.8],[71 28 28],[44 56 49.6 56 52.8 56 61 61],[39.2 33.6 32.8 33.6 40.8 33.6 30 12.4],[44 44 44 61 61],[28 71 60 66.4 90],[75 67 83 75 67 83 75 75],[54 42 42 54 54 54 54 66],[61 75 75],[24 24 42],[75 75 61],[66,76,76])
  VECT : Subsystem  mask(VECT){nb_p=4/4, lambda=0.192, freq_max=20e3, Ts_vect=60e-6, h=2}
      mask prompts: nb_p "Motor pairs of poles"; lambda "Flux induced by magnets (Wb)"; freq_max "Maximum switching frequency (Hz)"; Ts_vect "Sampling time (s)"; h "Current hysteresis bandwidth (A)"
      mask help: This block implements a vector controller.
      mask init:
      | load spsdrivelogodata.mat
      mask Display:
      | patch([spsdrivelogodata.X1 spsdrivelogodata.X1m],[spsdrivelogodata.Y1 spsdrivelogodata.Y1m],spsdrivelogodata.color1);
      | patch(spsdrivelogodata.X3,spsdrivelogodata.Y3,spsdrivelogodata.color2);
      | plot([spsdrivelogodata.X1 spsdrivelogodata.X1m spsdrivelogodata.X2 spsdrivelogodata.X2m spsdrivelogodata.X3 spsdrivelogodata.X4],[spsdrivelogodata.Y1 spsdrivelogodata.Y1m spsdrivelogodata.Y2 spsdrivelogodata.Y2m spsdrivelogodata.Y3 spsdrivelogodata.Y4]);
  + : PMIOPort  Side=Right
  - : PMIOPort  Port=2  Side=Right
  Gen_Sh : PMIOPort  Port=3  Side=Right
  wires:
  GF/1(Out1) -> VECT/1(Torque*)
  Subsystem1/1(Spd) -> Permanent Magnet Synchronous Machine/1
  Subsystem/1(Out) -> Subsystem1/1(Sig)
  Bus Selector/1 -> VECT/2(teta)  "<Rotor angle thetam (rad)>"
  Permanent Magnet Synchronous Machine/1 -> Mux/2(m), Bus Selector/1, Subsystem/1(In)
  TReq/1 -> GF/1(In1)
  Mux/1(Ctrl) -> Three-phase Inverter/1(ctrl)
  VECT/1(sig*) -> Mux/1(sig*)
  Measures/1(I_abc) -> VECT/3(I_abc)
  connections:
  Shaft Inertia/LConn1 -- Subsystem1/RConn1 -- Gen_Sh/RConn1
  Three-phase Inverter/LConn3 -- Measures/LConn3
  Measures/LConn2 -- Three-phase Inverter/LConn2
  Three-phase Inverter/LConn1 -- Measures/LConn1
  Measures/RConn3 -- Permanent Magnet Synchronous Machine/LConn3
  Measures/RConn2 -- Permanent Magnet Synchronous Machine/LConn2
  Measures/RConn1 -- Permanent Magnet Synchronous Machine/LConn1
  +/RConn1 -- Three-phase Inverter/RConn1
  -/RConn1 -- Three-phase Inverter/RConn2

== system HEV_Electrical_Lib/Mean Value/Synchronous Motor & Drive ==
  note: This block is based on the
      | AC6 IPMSM drive block
  TReq : Inport
  500 Vdc 50kW PMSM : spsPermanentMagnetSynchronousMachineLib/Permanent Magnet Synchronous Machine  NbPhases=3  FluxDistribution=Sinusoidal  RotorType=Salient-pole  MechanicalLoad=Speed w  PresetModel=No  ShowDetailedParameters=on  MeasurementBus=off  Resistance=HEV_Param.Motor.Stator_Resistance  Inductance=0  dqInductances=HEV_Param.Motor.Inductances  La=0.000835  MachineConstant=Flux linkage established by magnets (V.s)  Flux=0.175666143629361  VoltageCst=127.4493  TorqueCst=1.054  Flat=0  Mechanical=[0.089 0.005 4]  PolePairs=4  InitialConditions=[0,0,0,0]  InitialConditions5ph=[0 0 0 0 0 0]  RefAngle=90 degrees behind phase A axis (modified Park)  IterativeDiscreteModel=Trapezoidal non iterative  TsBlock=-1  TsPowergui=0
      settings: AttributesFormatString=\n
  Bus Selector : BusSelector  OutputSignals=Rotor speed wm (rad/s),Rotor angle thetam (rad)
  GF : Subsystem
      mask Display: disp('GF')
  Measures : Subsystem
      settings: LibrarySourceBlock=electricdrivelib/AC drives/PM Synchronous Motor Drive/Measures
  Mux : Subsystem
  Shaft Inertia : fl_lib/Mechanical/Rotational Elements/Inertia  inertia=HEV_Param.Motor.Shaft_Inertia kg*m^2  num_ports=foundation.enum.numPorts2.one  w_specify=on  w_priority=High  w=0 rad/s  w_nominal_specify=off  w_nominal_value=1  w_nominal_unit=rad/s  t_specify=off  t_priority=High  t=0 N*m  t_nominal_specify=off  t_nominal_value=1  t_nominal_unit=N*m
  Subsystem : Subsystem
      mask Display: disp('GF');
  Subsystem1 : Subsystem
  Three-phase Inverter : Subsystem  mask(SPSdrives Converter){Arms=3, SnubberResistance=5000, SnubberCapacitance=inf, Device=IGBT / Diodes, Ron=1e-3, Lon=0, ForwardVoltages=[0.8,0.8], ForwardVoltage=0, GTOparameters=[0,0], IGBTparameters=[1e-6,2e-6], Measurements=All voltages and currents, SourceFrequency=60, dqInductances=HEV_Param.Motor.Inductances, Flux=0.175666143629361, Resistance=HEV_Param.Motor.Stator_Resistance, p=4, converterType=Inverter}
      mask prompts: Arms "Number of bridge arms:"; SnubberResistance "Snubber resistance Rs (Ohms)"; SnubberCapacitance "Snubber capacitance Cs (F)"; Device "Power Electronic device"; Ron "Ron (Ohms)"; Lon "Lon (H)"; ForwardVoltages "Forward voltages  [ Device Vf(V) , Diode Vfd(V)]"; ForwardVoltage "Forward voltage Vf (V)"; GTOparameters "[  Tf (s) , Tt (s)  ]"; IGBTparameters "[  Tf (s) , Tt (s)  ]"; SourceFrequency "Source Frequency (Hz)"; dqInductances "PMSM-Inductances [ Ld(H) Lq(H) ]:"; Flux "PMSM-Flux induced by magnets (Wb):"; Resistance "PMSM-Stator resistance Rs (ohm):"; p "PMSM-Pairs of poles p:"; converterType "Converter type:"
      mask init:
      | Ld=dqInductances(1);
      | Lq=dqInductances(2);
      | Fcs=6*SourceFrequency/10;
      settings: OpenFcn=power_openblockproxy();
      mask Help: web(psbhelp);
      mask TypeOptions Arms: 1 | 2 | 3
      mask TypeOptions Device: Diodes | Thyristors | GTO / Diodes | MOSFET / Diodes | IGBT / Diodes | Ideal Switches
      mask TypeOptions Measurements: None | Device voltages | Device currents | UAB UBC UCA UDC voltages | All voltages and currents
      mask TypeOptions converterType: Rectifier | Inverter
      mask Display: plot(0,0,100,100,[39 39 23.8],[71 28 28],[44 56 49.6 56 52.8 56 61 61],[39.2 33.6 32.8 33.6 40.8 33.6 30 12.4],[44 44 44 61 61],[28 71 60 66.4 90],[75 67 83 75 67 83 75 75],[54 42 42 54 54 54 54 66],[61 75 75],[24 24 42],[75 75 61],[66,76,76])
  Torque limitation : Subsystem
      mask Display: plot([0;1800;2000;2500;3000;3500], [1;1;0.90*1;0.72*1;0.6*1;0.51*1])
  VECT controller : Subsystem  mask(VECT){nb_p=4, dqInductances=HEV_Param.Motor.Inductances, lambda=0.175666143629361, Ts_vect=60e-6}
      mask prompts: nb_p "Motor pairs of poles"; dqInductances "Inductances [ Ld(H) Lq(H) ]:"; lambda "Flux induced by magnets (Wb)"; Ts_vect "Sampling time (s)"
      mask help: This block implements a vector controller.
      mask init: same as HEV_Electrical_Lib/Detailed/Synchronous Motor & Drive/VECT Controller
      mask Display:
      | patch([spsdrivelogodata.X1 spsdrivelogodata.X1m],[spsdrivelogodata.Y1 spsdrivelogodata.Y1m],spsdrivelogodata.color1);
      | patch(spsdrivelogodata.X3,spsdrivelogodata.Y3,spsdrivelogodata.color2);
      | plot([spsdrivelogodata.X1 spsdrivelogodata.X1m spsdrivelogodata.X2 spsdrivelogodata.X2m spsdrivelogodata.X3 spsdrivelogodata.X4],[spsdrivelogodata.Y1 spsdrivelogodata.Y1m spsdrivelogodata.Y2 spsdrivelogodata.Y2m spsdrivelogodata.Y3 spsdrivelogodata.Y4]);
  + : PMIOPort  Side=Right
  - : PMIOPort  Port=2  Side=Right
  Mot_Sh : PMIOPort  Port=3  Side=Right
  wires:
  Subsystem/1(Motor) -> Subsystem1/1(Sig)
  Subsystem1/1(Spd) -> 500 Vdc 50kW PMSM/1
  GF/1(Out1) -> Torque limitation/2(Torque)
  TReq/1 -> GF/1(In1)
  Torque limitation/1(torque) -> VECT controller/1(Torque*)
  Bus Selector/2 -> VECT controller/3(teta)  "<Rotor angle thetam (rad)>"
  Measures/1(I_abc) -> VECT controller/4(I_abc)
  Bus Selector/1 -> Torque limitation/1(N rad/s), VECT controller/2(w)  "<Rotor speed wm (rad/s)>"
  500 Vdc 50kW PMSM/1 -> Subsystem/1(In1), Mux/2(m), Bus Selector/1
  VECT controller/1(sig*) -> Mux/1(sig*)
  Mux/1(Ctrl) -> Three-phase Inverter/1(ctrl)
  connections:
  Shaft Inertia/LConn1 -- Mot_Sh/RConn1 -- Subsystem1/RConn1
  -/RConn1 -- Three-phase Inverter/RConn2
  +/RConn1 -- Three-phase Inverter/RConn1
  Measures/RConn1 -- 500 Vdc 50kW PMSM/LConn1
  Measures/RConn2 -- 500 Vdc 50kW PMSM/LConn2
  Measures/RConn3 -- 500 Vdc 50kW PMSM/LConn3
  Three-phase Inverter/LConn1 -- Measures/LConn1
  Measures/LConn2 -- Three-phase Inverter/LConn2
  Three-phase Inverter/LConn3 -- Measures/LConn3

== system HEV_Electrical_Lib/Mean Value/Voltage Sensor1 ==
  V1 : spsVoltageMeasurementLib/Voltage Measurement  PhasorSimulation=off  OutputType=Complex  PSBequivalent=0
  + : PMIOPort  Tag=PMCPort  Side=Right
  - : PMIOPort  Port=2  Side=Left
  tag scope: DC_Bus_SYS=global
  wires:
  V1/1 -> [DC_Bus_SYS]
  connections:
  +/RConn1 -- V1/LConn1
  -/RConn1 -- V1/LConn2
